simulink model "youbot_predefinedpath_1405"  (R2024b)
settings: Solver=FixedStepAuto  StartTime=0.0  StopTime=inf  FixedStep=0.0001  RelTol=1e-3  EnableMultiTasking=on
values from neighbouring files (symbols this model uses):
  dt = (tf-ti)/n    (= 0.05)    [sss.m]    (also in youbotdynamiceqn.m = 0.1; youbotdynamiceqn_predefinedpath.m)
  Kdx = 1.5    [sss.m]    (also in youbotdynamiceqn_predefinedpath.m)
  Kdy = 1.5    [sss.m]    (also in youbotdynamiceqn_predefinedpath.m)
  Kdz = 0.001    [sss.m]    (also in youbotdynamiceqn_predefinedpath.m = 2.5)
  Kpx = 1.5    [sss.m]    (also in youbotdynamiceqn_predefinedpath.m)
  Kpy = 1.5    [sss.m]    (also in youbotdynamiceqn_predefinedpath.m)
  Kpz = 0.005    [sss.m]    (also in youbotdynamiceqn_predefinedpath.m = 2.5)
  M_r = [m  0  0 ... (first row only)    [sss.m]    (also in youbotdynamiceqn.m; youbotdynamiceqn_predefinedpath.m)
  M_w = diag([I_w1, I_w2, I_w3, I_w4])    [sss.m]    (also in youbotdynamiceqn.m; youbotdynamiceqn_predefinedpath.m)
  R = (1/r) * [  1, -1, -(L+l) ... (first row only)    [sss.m]    (also in youbotdynamiceqn.m; youbotdynamiceqn_predefinedpath.m)
  R_T = transpose(R)    [sss.m]    (also in youbotdynamiceqn.m; youbotdynamiceqn_predefinedpath.m)
  waypoint = zeros(size(pathObj.States, 1),2)    [astar.m]    (also in rrt-son.m; rrt.m; rrtson.m)
undefined symbols (not defined in the file or in its folder): Angular, DiscIntNeverNeededParam, Linear
libraries: robotlib x3, slpidlib x1
settings Model: PacingRate=0.790000  Creator=The MathWorks, Inc.  LastModifiedBy=a_met
settings SolverCC: AutoInsertRateTranBlk=on
settings DataIOCC: LimitDataPoints=on  SaveFormat=Array  ReturnWorkspaceOutputs=off
settings OptimizationCC: ZeroExternalMemoryAtStartup=off  ZeroInternalMemoryAtStartup=off  LifeSpan=1  MaxStackSize=64
settings DebuggingCC: AlgebraicLoopMsg=none  SolverPrmCheckMsg=warning  UnconnectedInputMsg=warning  UnconnectedOutputMsg=warning  UnconnectedLineMsg=warning  SFUnexpectedBacktrackingDiag=warning  SFNoUnconditionalDefaultTransitionDiag=warning  SFExecutionAtInitializationDiag=none  ArithmeticOperatorsInVariantConditions=warning
settings HardwareCC: ProdBitPerPointer=32  ProdBitPerSizeT=32  ProdBitPerPtrDiffT=32  ProdLargestAtomicFloat=None  ProdIntDivRoundTo=Undefined  ProdEndianess=Unspecified  ProdWordSize=32  ProdHWDeviceType=Generic->Unspecified (assume 32-bit Generic)  TargetHWDeviceType=Generic->Unspecified (assume 32-bit Generic)  UseEmbeddedCoderFeatures=off
settings ModelReferenceCC: EnableRefExpFcnMdlSchedulingChecks=on  PropagateSignalLabelsOutOfModel=off
settings SFSimCC: SimUseLocalCustomCode=off  CustomCodeUndefinedFunction=UseInterfaceOnly  SimTargetLang=C++
settings RTWCC: Description=Embedded Coder  SystemTargetFile=ert.tlc  HardwareBoard=Robot Operating System (ROS)  TLCOptions=-aInlineSetEventsForThisBaseRateFcn=TLC_FALSE -aSuppressMultiTaskScheduler=TLC_FALSE -aRateBasedStepFcn=0  TemplateMakefile=ert_default_tmf  RTWUseLocalCustomCode=off  Toolchain=Catkin  TargetLang=C++  GPUComputeCapability=3.5
settings CodeAppCC: StateflowObjectComments=on
settings ERTTargetCC: MultiwordLength=2048  ERTCustomFileBanners=off  CodeInterfacePackaging=C++ class  SupportContinuousTime=on  SupportNonInlinedSFcns=on  RemoveResetFunc=off  SupportVariableSizeSignals=on  ModelStepFunctionPrototypeControlCompliant=off  InlinedParameterPlacement=Hierarchical  RootIOFormat=Structure reference  ConvertIfToSwitch=off  SuppressUnreachableDefaultCases=off  DynamicArrayContainerType=coder::array
settings ConfigComp: CovMetricSettings=dw  CovSaveCumulativeToWorkspaceVar=on  CovSaveSingleToWorkspaceVar=on  CovExternalEMLEnable=off  CovSFcnEnable=off

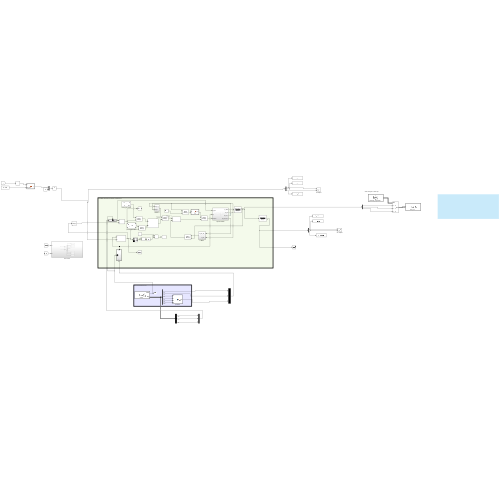
[thumbnail: Simulink's stored preview of the top-level diagram]
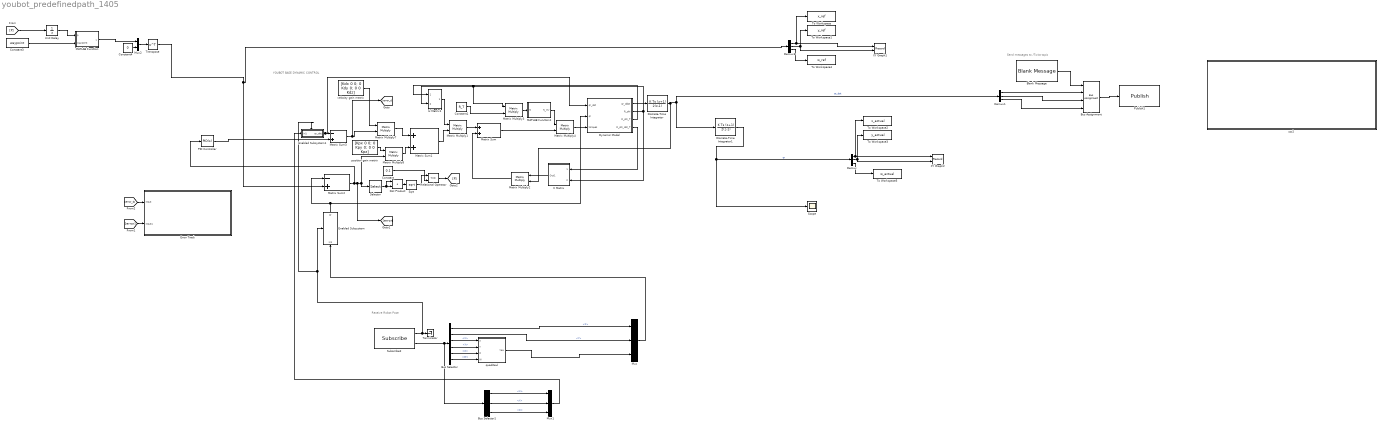
== system youbot_predefinedpath_1405 ==
  note: YOUBOT BASE DYNAMIC CONTROL
  note: Send messages to /Twist topic
  note: Receive Robot Pose
  Blank Message : robotlib/Blank Message  messageClass=Message  entityType=geometry_msgs/Twist  messageType=geometry_msgs/Twist  SampleTime=inf  legacyBusStruct=off
  Bus Assignment : BusAssignment  AssignedSignals=Linear.X,Linear.Y,Angular.Z
  Bus Selector : BusSelector  OutputSignals=Pose.Pose.Position.X,Pose.Pose.Position.Y,Pose.Pose.Orientation.X,Pose.Pose.Orientation.Y,Pose.Pose.Orientation.Z,Pose.Pose.Orientation.W
  Bus Selector1 : BusSelector  OutputSignals=Twist.Twist.Linear.X,Twist.Twist.Linear.Y,Twist.Twist.Angular.Z
  Constant : Constant  Value=0.1
  Constant1 : Constant  Value=R_T
  Constant3 : Constant  Value=waypoint
  Constant4 : Constant  Value=0
  Demux : Demux  Outputs=3
  Demux1 : Demux  Outputs=3
  Demux3 : Demux  Outputs=3
  Discrete-Time Integrator : DiscreteIntegrator  IntegratorMethod=Integration: Trapezoidal  SampleTime=-1  ICPrevOutput=DiscIntNeverNeededParam  ICPrevScaledInput=DiscIntNeverNeededParam
  Discrete-Time Integrator1 : DiscreteIntegrator  IntegratorMethod=Integration: Trapezoidal  SampleTime=-1  ICPrevOutput=DiscIntNeverNeededParam  ICPrevScaledInput=DiscIntNeverNeededParam
  Dot Product : DotProduct  OutDataTypeStr=Inherit: Inherit via internal rule
  Dynamic Model : Subsystem
  Enabled Subsystem : Subsystem  TreatAsAtomicUnit=on
  Enabled Subsystem1 : Subsystem  TreatAsAtomicUnit=on
  Error Track : Subsystem
  H Matrix1 : Subsystem
  K Matrix : Subsystem
  MATLAB Function : MATLAB Function  TreatAsAtomicUnit=on
  MATLAB Function1 : MATLAB Function  TreatAsAtomicUnit=on
  Matrix Sum : Sum
  Matrix Sum1 : Sum
  Matrix Sum2 : Sum  Inputs=-+
  Matrix Sum3 : Sum  Inputs=-+
  Matrix Multiply1 : Product  Multiplication=Matrix(*)  SampleTime=dt
  Matrix Multiply{2..4,7..8} (5 alike) : Product  Multiplication=Matrix(*)
  Mux : Mux  Inputs=3
  Mux1 : Mux  Inputs=3
  Mux2 : Mux  Inputs=2
  PID Controller : slpidlib/PID Controller  Controller=PID  Form=Parallel  TimeDomain=Continuous-time  UseExternalTs=off  SampleTime=-1  IntegratorMethod=Forward Euler  FilterMethod=Forward Euler  ControllerParametersSource=internal  P=0.02  I=0  UseKiTs=off  D=0  UseExternalDerivativeSource=off  N=100  UseFilter=on  TunerSelectOption=Transfer Function Based (PID Tuner App)  InitialConditionSource=internal  InitialConditionForIntegrator=0  InitialConditionForFilter=0  DifferentiatorICPrevScaledInput=0  ExternalReset=none  TrackingMode=off  Kt=1  LimitOutput=off  SatLimitsSource=internal  UpperSaturationLimit=inf  LowerSaturationLimit=-inf  LinearizeAsGain=on  AntiWindupMode=none  Kb=1  LimitIntegrator=off  UpperIntegratorSaturationLimit=inf  LowerIntegratorSaturationLimit=-inf  POutMin=[]  POutMax=[]  IOutMin=[]  IOutMax=[]  DOutMin=[]  DOutMax=[]  NOutMin=[]  NOutMax=[]  SumOutMin=[]  SumOutMax=[]  SaturationOutMin=[]  SaturationOutMax=[]  PParamMin=[]  PParamMax=[]  IParamMin=[]  IParamMax=[]  DParamMin=[]  DParamMax=[]  NParamMin=[]  NParamMax=[]  KbParamMin=[]  KbParamMax=[]  KtParamMin=[]  KtParamMax=[]  KbOutMin=[]  KbOutMax=[]  KtOutMin=[]  KtOutMax=[]  IntegratorOutMin=[]  IntegratorOutMax=[]  FilterOutMin=[]  FilterOutMax=[]  SumI1OutMin=[]  SumI1OutMax=[]  SumI2OutMin=[]  SumI2OutMax=[]  SumI3OutMin=[]  SumI3OutMax=[]  SumI4OutMin=[]  SumI4OutMax=[]  SumDOutMin=[]  SumDOutMax=[]  DifferentiatorOutMin=[]  DifferentiatorOutMax=[]  FilterDiffOutCoefMin=[]  FilterDiffOutCoefMax=[]  ReciprocalOutMin=[]  ReciprocalOutMax=[]  SumDenOutMin=[]  SumDenOutMax=[]  SumNumOutMin=[]  SumNumOutMax=[]  DivideOutMin=[]  DivideOutMax=[]  UdiffTsProdOutMin=[]  UdiffTsProdOutMax=[]  NTsProdOutMin=[]  NTsProdOutMax=[]  UintegralTsProdOutMin=[]  UintegralTsProdOutMax=[]  UngainTsProdOutMin=[]  UngainTsProdOutMax=[]  ClampingZeroOutDataTypeStr=Inherit: Inherit via back propagation  ClampingZeroOutMin=[]  ClampingZeroOutMax=[]  FilterDenConstantOutDataTypeStr=Inherit: Inherit via back propagation  FilterDenConstantOutMin=[]  FilterDenConstantOutMax=[]  PCopyOutDataTypeStr=Inherit: Inherit via back propagation  PCopyOutMin=[]  PCopyOutMax=[]  NCopyOutDataTypeStr=Inherit: Inherit via back propagation  NCopyOutMin=[]  NCopyOutMax=[]  IntegratorContinuousStateAttributes=''  IntegratorStateMustResolveToSignalObject=off  IntegratorRTWStateStorageClass=Auto  FilterContinuousStateAttributes=''  FilterStateMustResolveToSignalObject=off  FilterRTWStateStorageClass=Auto  ParallelPVariant=InternalParameters  IdealPVariant=Disabled  IVariant=InternalParameters  DVariant=InternalParameters  IntegratorVariant=Continuous  SatVariant=Disabled  AWVariant=Passthrough  PCopyVariant=Disabled  TRVariant=Disabled  FdbkBlocksVariant=Forward  IdealPFdbkVariant=Disabled  SatFdbkVariant=Disabled  DerivativeFilterVariant=ContFilter  NVariant=InternalParameters  NCopyVariant=Disabled  FilterICVariant=InternalICsFilter  IntegratorICVariant=InternalICs  ExternalResetVariant=Disabled  TRSumVariant=Passthrough  SumFdbkVariant=Disabled  SumVariant=Sum_PID  TsampFilterVariant=InternalTs  TsampNgainVariant=Passthrough  TsampIntegralVariant=Disabled_SignalSpec  ExternalSaturationOutDataTypeStr=Inherit: Same as second input  DerivativeSourceVariant=ErrorSignal  PreIntVariant=InternalPreInt
  Publish1 : robotlib/Publish  topicSource=Select from ROS network  topic=/cmd_vel  messageType=geometry_msgs/Twist  legacyBusStruct=off  messageQueueLength=105
  Relational Operator : RelationalOperator  Operator=<=  OutDataTypeStr=boolean  RndMeth=Simplest  InputSameDT=off
  Scope : Scope
  Selector : Selector  InputPortWidth=3  IndexOptions=Index vector (dialog)  Indices=[1 2]  OutputSizes=1
  Sqrt : Sqrt
  Subscribe2 : robotlib/Subscribe  topicSource=Select from ROS network  topic=/odom  messageType=nav_msgs/Odometry  SampleTime=-1  legacyBusStruct=off  messageQueueLength=1
  Terminator : Terminator
  To Workspace : ToWorkspace  VariableName=x_ref  SaveFormat=Timeseries  SampleTime=-1
  To Workspace1 : ToWorkspace  VariableName=y_ref  SaveFormat=Timeseries  SampleTime=-1
  To Workspace2 : ToWorkspace  VariableName=x_actual  SaveFormat=Timeseries  SampleTime=-1
  To Workspace3 : ToWorkspace  VariableName=y_actual  SaveFormat=Timeseries  SampleTime=-1
  To Workspace4 : ToWorkspace  VariableName=w_ref  SaveFormat=Timeseries  SampleTime=-1
  To Workspace5 : ToWorkspace  VariableName=w_actual  SaveFormat=Timeseries  SampleTime=-1
  Transpose : Math  Operator=transpose
  Unit Delay : UnitDelay  SampleTime=-1  HasFrameUpgradeWarning=on
  XY Graph1 : Record  FileSettingsInternal="{\"entries\":[{\"content\":{\"excelSettings\":{\"content\":{},\"type\":\"Streamout.ExcelSettings\"}},\"type\":\"Streamout.FileSettingStorage\",\"uuid\":\"\"}],\"packageUris\":[\"http:\\/\\/schema.mathworks.com\\/mf0\\/streamout_blocks\\/R2020a\"],\"version\":\"1.0\"}"  Layout=[1 1]  SignalsInternal="{\"entries\":[{\"content\":{\"signals\":[{\"content\":{\"blockPath\":[],\"dimensions\":[1,1],\"domain\":\"\",\"lineColor\":\"#a2142f\",\"plots\":[ 1 ],\"port\":1,\"sid\":[\"\"],\"signalID\":1,\"signalName\":\"Demux3:1\"},\"type\":\"RecordBlkView.Signal\",\"uuid\":\"\"},{\"content\":{\"blockPath\":[],\"dimensions\":[1,1],\"domain\":\"\",\"lineColor\":\"#139fff\",\"plots\":[ 1 ],\"port\":2,\"sid\":[\"\"],\"signalID\":2,\"signalName\":\"Demux3:2\"},\"type\":\"RecordBlkView.Signal\",\"uuid\":\"\"}]},\"type\":\"RecordBlkView.InputSignals\",\"uuid\":\"\"}],\"packageUris\":[\"http:\\/\\/schema.mathworks.com\\/mf0\\/streamout_blocks\\/R2020a\"],\"version\":\"1.0\"}"  VisualizationBindings="{\"xyplotplugin\":{\"info\":[{\"series\":[{\"bindingParametersList\":[{\"parameter\":\"X-Axis\",\"signalID\":1,\"signalName\":\"Demux3:1\"},{\"parameter\":\"Y-Axis\",\"signalID\":2,\"signalName\":\"Demux3:2\"}],\"seriesID\":0}],\"subplotID\":1}]}}"  CompatibilityTag=XY
  XY Graph2 : Record  FileSettingsInternal="{\"entries\":[{\"content\":{\"excelSettings\":{\"content\":{},\"type\":\"Streamout.ExcelSettings\"}},\"type\":\"Streamout.FileSettingStorage\",\"uuid\":\"\"}],\"packageUris\":[\"http:\\/\\/schema.mathworks.com\\/mf0\\/streamout_blocks\\/R2020a\"],\"version\":\"1.0\"}"  Layout=[1 1]  SignalsInternal="{\"entries\":[{\"content\":{\"signals\":[{\"content\":{\"blockPath\":[],\"dimensions\":[1,1],\"domain\":\"\",\"lineColor\":\"#a2142f\",\"plots\":[ 1 ],\"port\":1,\"sid\":[\"\"],\"signalID\":1,\"signalName\":\"Demux:1\"},\"type\":\"RecordBlkView.Signal\",\"uuid\":\"\"},{\"content\":{\"blockPath\":[],\"dimensions\":[1,1],\"domain\":\"\",\"lineColor\":\"#139fff\",\"plots\":[ 1 ],\"port\":2,\"sid\":[\"\"],\"signalID\":2,\"signalName\":\"Demux:2\"},\"type\":\"RecordBlkView.Signal\",\"uuid\":\"\"}]},\"type\":\"RecordBlkView.InputSignals\",\"uuid\":\"\"}],\"packageUris\":[\"http:\\/\\/schema.mathworks.com\\/mf0\\/streamout_blocks\\/R2020a\"],\"version\":\"1.0\"}"  VisualizationBindings="{\"xyplotplugin\":{\"info\":[{\"series\":[{\"bindingParametersList\":[{\"parameter\":\"X-Axis\",\"signalID\":1,\"signalName\":\"Demux:1\"},{\"parameter\":\"Y-Axis\",\"signalID\":2,\"signalName\":\"Demux:2\"}],\"seriesID\":0}],\"subplotID\":1}]}}"  CompatibilityTag=XY
  position gain matrix : Constant  Value=[Kpx 0 0; 0 Kpy 0; 0 0 Kpz]
  quad2eul : MATLAB Function  TreatAsAtomicUnit=on
  velocity gain matrix : Constant  Value=[Kdx 0 0; 0 Kdy 0; 0 0 Kdz]
  zzz1 : Subsystem  TreatAsAtomicUnit=on
      settings: OpenFcn=% no-op
      mask Display: disp('')
  wires:
  Demux/1 -> To Workspace2/1, XY Graph2/1
  Demux/2 -> XY Graph2/2, To Workspace3/1
  Demux3/2 -> XY Graph1/2, To Workspace1/1
  Demux3/1 -> To Workspace/1, XY Graph1/1
  Dynamic Model/1(qr_ddot) -> Discrete-Time Integrator/1
  Matrix Multiply4/1 -> Dynamic Model/3(torques)
  Matrix Multiply2/1 -> Matrix Sum/2
  K Matrix/1(Out1) -> Matrix Multiply2/1
  Matrix Multiply7/1 -> Matrix Sum1/1
  Matrix Multiply3/1 -> MATLAB Function1/1(N)
  Matrix Sum1/1 -> Matrix Multiply1/2
  H Matrix1/1(Out1) -> Matrix Multiply1/1
  Constant1/1 -> Matrix Multiply3/2
  Dynamic Model/4(R_phi_dot_T) -> K Matrix/1(R_phi_dot_T)
  MATLAB Function1/1(N_inv) -> Matrix Multiply4/1
  Dynamic Model/3(R_phi_T) -> H Matrix1/1(R_phi_T)
  Matrix Sum3/1 -> Matrix Multiply7/2, [error_d]
  Discrete-Time Integrator/1 -> Demux1/1, Discrete-Time Integrator1/1, Matrix Multiply2/2  "qr_dot"
  Matrix Sum2/1 -> PID Controller/1, [error], Matrix Multiply8/2, Selector/1
  position gain matrix/1 -> Matrix Multiply8/1
  Dynamic Model/2(R_phi) -> K Matrix/2(R_phi_T), Matrix Multiply3/1, H Matrix1/2(R_phi)
  Matrix Multiply1/1 -> Matrix Sum/1
  Matrix Sum/1 -> Matrix Multiply4/2
  Matrix Multiply8/1 -> Matrix Sum1/2
  velocity gain matrix/1 -> Matrix Multiply7/1
  Discrete-Time Integrator1/1 -> Demux/1, Scope/1  "qr"
  Demux3/3 -> To Workspace4/1
  Demux/3 -> To Workspace5/1
  Mux2/1 -> Transpose/1
  [error] -> Error Track/2(Input1)
  [error_d] -> Error Track/1(Input)
  Demux1/3 -> Bus Assignment/4
  Demux1/2 -> Bus Assignment/3
  Bus Assignment/1 -> Publish1/1
  Blank Message/1 -> Bus Assignment/1
  Demux1/1 -> Bus Assignment/2
  Bus Selector/2 -> Mux/2  "<Y>"
  Bus Selector/3 -> quad2eul/1(X)  "<X>"
  quad2eul/1(Yaw) -> Mux/3
  Bus Selector/1 -> Mux/1  "<X>"
  Bus Selector/5 -> quad2eul/3(Z)  "<Z>"
  Subscribe2/2 -> Bus Selector1/1, Bus Selector/1
  Bus Selector/6 -> quad2eul/4(W)  "<W>"
  Subscribe2/1 -> Enabled Subsystem1/Enable, Enabled Subsystem/Enable, Terminator/1
  Bus Selector/4 -> quad2eul/2(Y)  "<Y>"
  Mux/1 -> Enabled Subsystem/1(In1)
  Enabled Subsystem/1(qr) -> Dynamic Model/2(qr), Matrix Sum2/1
  Bus Selector1/1 -> Mux1/1  "<X>"
  Bus Selector1/2 -> Mux1/2  "<Y>"
  Bus Selector1/3 -> Mux1/3  "<Z>"
  Enabled Subsystem1/1(qr_dot) -> Dynamic Model/1(qr_dot), Matrix Sum3/1
  Mux1/1 -> Enabled Subsystem1/1(In1)
  PID Controller/1 -> Matrix Sum3/2
  Relational Operator/1 -> [P]
  Selector/1 -> Dot Product/1, Dot Product/2
  Dot Product/1 -> Sqrt/1
  Constant3/1 -> MATLAB Function/2(waypoint)
  MATLAB Function/1(y) -> Mux2/1
  Constant4/1 -> Mux2/2
  Transpose/1 -> Matrix Sum2/2, Demux3/1
  Sqrt/1 -> Relational Operator/1
  Constant/1 -> Relational Operator/2
  [P] -> Unit Delay/1
  Unit Delay/1 -> MATLAB Function/1(p)

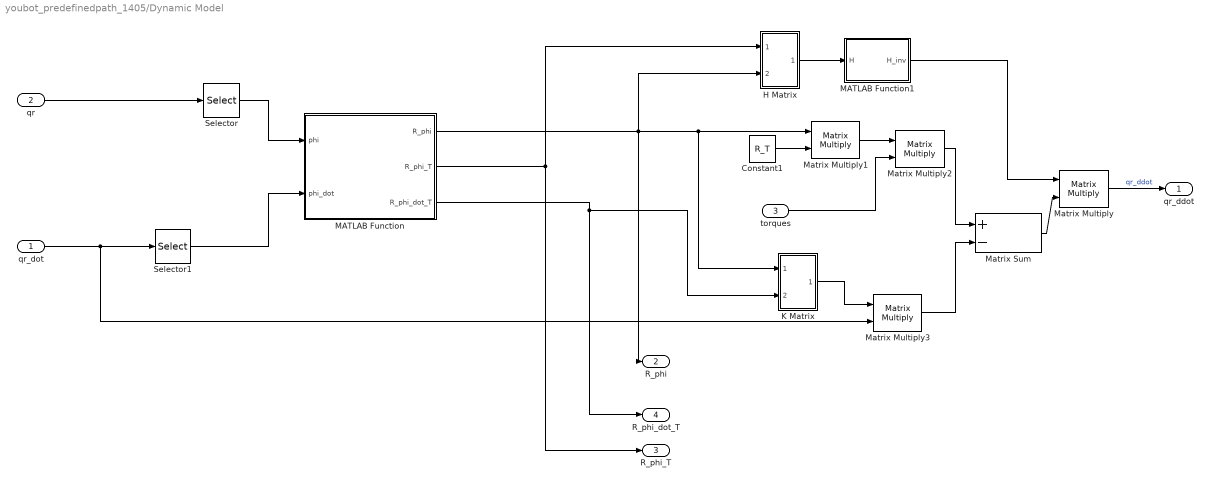
== system youbot_predefinedpath_1405/Dynamic Model ==
  qr_dot : Inport
  qr : Inport  Port=2
  torques : Inport  Port=3
  Constant1 : Constant  Value=R_T
  H Matrix : Subsystem
  K Matrix : Subsystem
  MATLAB Function : MATLAB Function  TreatAsAtomicUnit=on
  MATLAB Function1 : MATLAB Function  TreatAsAtomicUnit=on
  Matrix Sum : Sum  Inputs=+-
  Matrix Multiply{,1..3} (4 alike) : Product  Multiplication=Matrix(*)
  Selector : Selector  InputPortWidth=3  IndexOptions=Index vector (dialog)  Indices=[3]  OutputSizes=1
  Selector1 : Selector  InputPortWidth=3  IndexOptions=Index vector (dialog)  Indices=[3]  OutputSizes=1
  qr_ddot : Outport  PortDimensions=[3 1]
  R_phi : Outport  Port=2
  R_phi_T : Outport  Port=3
  R_phi_dot_T : Outport  Port=4
  wires:
  torques/1 -> Matrix Multiply2/2
  MATLAB Function/3(R_phi_dot_T) -> R_phi_dot_T/1, K Matrix/2(R_phi_dot_T)
  MATLAB Function/2(R_phi_T) -> R_phi_T/1, H Matrix/1(In2)
  Matrix Multiply2/1 -> Matrix Sum/1
  Matrix Multiply3/1 -> Matrix Sum/2
  K Matrix/1(Out1) -> Matrix Multiply3/1
  MATLAB Function1/1(H_inv) -> Matrix Multiply/1
  MATLAB Function/1(R_phi) -> K Matrix/1(R_phi), Matrix Multiply1/1, R_phi/1, H Matrix/2(In1)
  Constant1/1 -> Matrix Multiply1/2
  Matrix Multiply1/1 -> Matrix Multiply2/1
  Matrix Multiply/1 -> qr_ddot/1  "qr_ddot"
  Matrix Sum/1 -> Matrix Multiply/2
  H Matrix/1(Out1) -> MATLAB Function1/1(H)
  Selector/1 -> MATLAB Function/1(phi)
  Selector1/1 -> MATLAB Function/2(phi_dot)
  qr/1 -> Selector/1
  qr_dot/1 -> Matrix Multiply3/2, Selector1/1

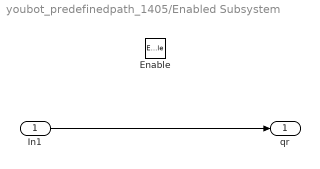
== system youbot_predefinedpath_1405/Enabled Subsystem ==
  In1 : Inport
  Enable : EnablePort
  qr : Outport
  wires:
  In1/1 -> qr/1

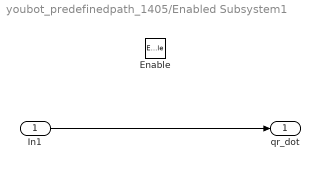
== system youbot_predefinedpath_1405/Enabled Subsystem1 ==
  In1 : Inport
  Enable : EnablePort
  qr_dot : Outport
  wires:
  In1/1 -> qr_dot/1

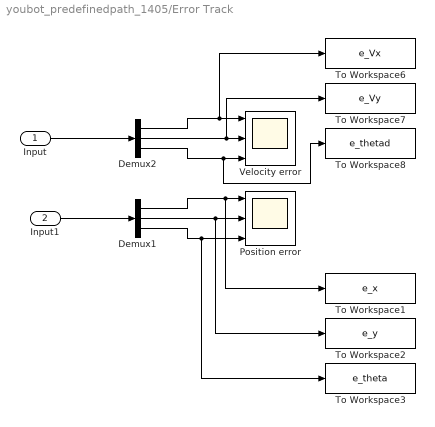
== system youbot_predefinedpath_1405/Error Track ==
  Input : Inport
  Input1 : Inport  Port=2
  Demux1 : Demux  Outputs=3
  Demux2 : Demux  Outputs=3
  Position error : Scope  NumInputPorts=3
  To Workspace1 : ToWorkspace  VariableName=e_x  SaveFormat=Timeseries  SampleTime=-1
  To Workspace2 : ToWorkspace  VariableName=e_y  SaveFormat=Timeseries  SampleTime=-1
  To Workspace3 : ToWorkspace  VariableName=e_theta  SaveFormat=Timeseries  SampleTime=-1
  To Workspace6 : ToWorkspace  VariableName=e_Vx  SaveFormat=Timeseries  SampleTime=-1
  To Workspace7 : ToWorkspace  VariableName=e_Vy  SaveFormat=Timeseries  SampleTime=-1
  To Workspace8 : ToWorkspace  VariableName=e_thetad  SaveFormat=Timeseries  SampleTime=-1
  Velocity error : Scope  NumInputPorts=3
  wires:
  Input1/1 -> Demux1/1
  Demux2/3 -> To Workspace8/1, Velocity error/3
  Demux1/1 -> To Workspace1/1, Position error/1
  Input/1 -> Demux2/1
  Demux1/2 -> To Workspace2/1, Position error/2
  Demux2/2 -> To Workspace7/1, Velocity error/2
  Demux1/3 -> To Workspace3/1, Position error/3
  Demux2/1 -> To Workspace6/1, Velocity error/1

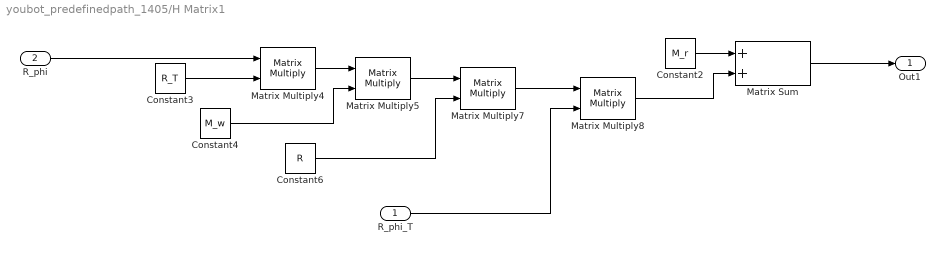
== system youbot_predefinedpath_1405/H Matrix1 ==
  R_phi_T : Inport
  R_phi : Inport  Port=2
  Constant2 : Constant  Value=M_r
  Constant3 : Constant  Value=R_T
  Constant4 : Constant  Value=M_w
  Constant6 : Constant  Value=R
  Matrix Sum : Sum
  Matrix Multiply{4..5,7..8} (4 alike) : Product  Multiplication=Matrix(*)  SampleTime=dt
  Out1 : Outport
  wires:
  Constant2/1 -> Matrix Sum/1
  Matrix Multiply4/1 -> Matrix Multiply5/1
  R_phi_T/1 -> Matrix Multiply8/2
  Matrix Multiply7/1 -> Matrix Multiply8/1
  Constant6/1 -> Matrix Multiply7/2
  Matrix Multiply8/1 -> Matrix Sum/2
  Constant4/1 -> Matrix Multiply5/2
  Constant3/1 -> Matrix Multiply4/2
  Matrix Sum/1 -> Out1/1
  Matrix Multiply5/1 -> Matrix Multiply7/1
  R_phi/1 -> Matrix Multiply4/1

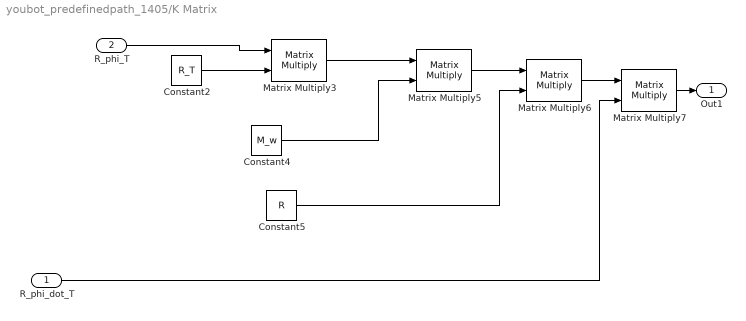
== system youbot_predefinedpath_1405/K Matrix ==
  R_phi_dot_T : Inport
  R_phi_T : Inport  Port=2
  Constant2 : Constant  Value=R_T
  Constant4 : Constant  Value=M_w
  Constant5 : Constant  Value=R
  Matrix Multiply{3,5..7} (4 alike) : Product  Multiplication=Matrix(*)
  Out1 : Outport  PortDimensions=[3 3]
  wires:
  Matrix Multiply7/1 -> Out1/1
  Matrix Multiply6/1 -> Matrix Multiply7/1
  Matrix Multiply3/1 -> Matrix Multiply5/1
  R_phi_T/1 -> Matrix Multiply3/1
  Constant4/1 -> Matrix Multiply5/2
  Constant5/1 -> Matrix Multiply6/2
  R_phi_dot_T/1 -> Matrix Multiply7/2
  Constant2/1 -> Matrix Multiply3/2
  Matrix Multiply5/1 -> Matrix Multiply6/1

== system youbot_predefinedpath_1405/zzz1 ==

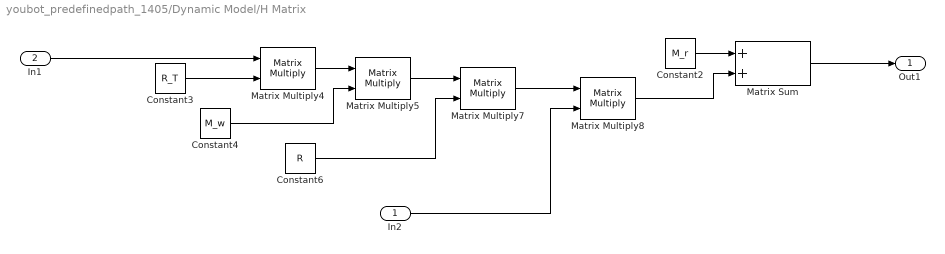
== system youbot_predefinedpath_1405/Dynamic Model/H Matrix ==
  In2 : Inport
  In1 : Inport  Port=2
  Constant2 : Constant  Value=M_r
  Constant3 : Constant  Value=R_T
  Constant4 : Constant  Value=M_w
  Constant6 : Constant  Value=R
  Matrix Sum : Sum
  Matrix Multiply{4..5,7..8} (4 alike) : Product  Multiplication=Matrix(*)
  Out1 : Outport
  wires:
  In1/1 -> Matrix Multiply4/1
  Matrix Multiply5/1 -> Matrix Multiply7/1
  Matrix Sum/1 -> Out1/1
  Constant3/1 -> Matrix Multiply4/2
  Constant4/1 -> Matrix Multiply5/2
  Matrix Multiply8/1 -> Matrix Sum/2
  Constant6/1 -> Matrix Multiply7/2
  Matrix Multiply7/1 -> Matrix Multiply8/1
  In2/1 -> Matrix Multiply8/2
  Matrix Multiply4/1 -> Matrix Multiply5/1
  Constant2/1 -> Matrix Sum/1

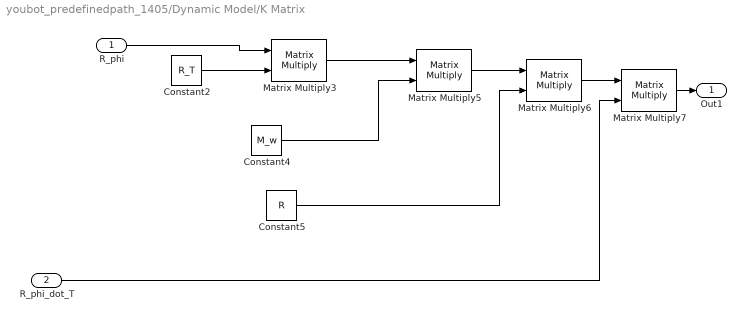
== system youbot_predefinedpath_1405/Dynamic Model/K Matrix ==
  R_phi : Inport
  R_phi_dot_T : Inport  Port=2
  Constant2 : Constant  Value=R_T
  Constant4 : Constant  Value=M_w
  Constant5 : Constant  Value=R
  Matrix Multiply{3,5..7} (4 alike) : Product  Multiplication=Matrix(*)
  Out1 : Outport
  wires:
  Matrix Multiply7/1 -> Out1/1
  Matrix Multiply6/1 -> Matrix Multiply7/1
  Matrix Multiply3/1 -> Matrix Multiply5/1
  R_phi/1 -> Matrix Multiply3/1
  Constant4/1 -> Matrix Multiply5/2
  Constant5/1 -> Matrix Multiply6/2
  R_phi_dot_T/1 -> Matrix Multiply7/2
  Constant2/1 -> Matrix Multiply3/2
  Matrix Multiply5/1 -> Matrix Multiply6/1

== matlab function youbot_predefinedpath_1405/Dynamic Model/MATLAB Function1 ==
  data: H input; H_inv output
function H_inv = fcn(H)

H_inv = inv(H);

== matlab function youbot_predefinedpath_1405/Dynamic Model/MATLAB Function ==
  data: phi input; R_phi output size=[3 3]; phi_dot input; R_phi_T output size=[3 3]; R_phi_dot_T output size=[3 3]
function [R_phi, R_phi_T, R_phi_dot_T] = fcn(phi, phi_dot)

    % Giriş değerlerini göster
    fprintf('phi: %f\n', phi);
    fprintf('phi_dot: %f\n', phi_dot);

    % NaN kontrolü
    if isnan(phi)
        warning('phi is NaN');
    end
    if isnan(phi_dot)
        warning('phi_dot is NaN');
    end

    R_phi = [ cos(phi), -sin(phi), 0;
              sin(phi),  cos(phi), 0;
                    0  ,        0 , 1];

    R_phi_dot = [ -sin(phi)*phi_dot, -cos(phi)*phi_dot, 0;
                   cos(phi)*phi_dot,  -sin(phi)*phi_dot, 0;
                             0      ,              0    , 0];

    % R_phi_dot matrisindeki NaN'leri kontrol et
    if any(isnan(R_phi_dot), 'all')
        warning('R_phi_dot contains NaN values');
        disp('R_phi_dot matrix:');
        disp(R_phi_dot);
    end
   if isnan(phi) || isnan(phi_dot)
    disp('phi or phi_dot is NaN at this timestep!');
    disp(sprintf('phi = %f', phi));
    disp(sprintf('phi_dot = %f', phi_dot));
    end
    R_phi_T = transpose(R_phi);
    R_phi_dot_T = transpose(R_phi_dot);

    % Sonuçları göster
    disp('R_phi_dot_T:');
    disp(R_phi_dot_T);

end

== matlab function youbot_predefinedpath_1405/MATLAB Function1 ==
  data: N input; N_inv output
function N_inv = fcn(N)

N_inv = pinv(N);

== matlab function youbot_predefinedpath_1405/quad2eul ==
  data: X input; Yaw output; Y input; Z input; W input
function Yaw = quat2eulBlk(X, Y, Z, W)
%#codegen

eularAngles = quat2eul([W, X, Y, Z]);
Yaw = eularAngles(1);

== matlab function youbot_predefinedpath_1405/MATLAB Function ==
  data: p input; y output; waypoint input
function y = fcn(p, waypoint)
% Her p değişiminde x + 1
persistent x p_prev

% İlk değerleri başlat
if isempty(x)
    x = 1; % Başlangıç değeri
end
if isempty(p_prev)
    p_prev = p;
end

% p değiştiyse (fark varsa)
if p ~= p_prev
    x = x + 1;
end

% p'nin son değerini güncelle
p_prev = p;

% Sınır kontrolü: x geçerli bir indeks mi?
x_safe = min(max(1, x), size(waypoint,1));

% İlgili satırı döndür
y = waypoint(x_safe,:);
